simulink library "speedgoatlib_fpga_analog_io"  (R2024b)
settings: Solver=VariableStepAuto  StartTime=0.0  StopTime=10.0  RelTol=1e-3
undefined symbols (not defined in the file): IO336, sg_fpga_callBackInit_m_a1, sg_fpga_io324_analog_input_m, sg_fpga_io324_analog_output_m, sg_fpga_io324_analog_setup_m, sg_fpga_io325_analog_input_m, sg_fpga_io325_analog_output_m, sg_fpga_io325_analog_setup_m, sg_fpga_io334_analog_input_m, sg_fpga_io334_analog_output_m, sg_fpga_io334_analog_setup_m, sg_fpga_io336_analog_input_m, sg_fpga_io336_analog_output_m, sg_fpga_io336_analog_setup_m, sg_fpga_io337_analog_input_m, sg_fpga_io337_analog_output_m, sg_fpga_io337_analog_setup_m, sg_fpga_io3xx_120_analog_input_m, sg_fpga_io3xx_120_analog_output_m, sg_fpga_io3xx_120_analog_setup_m
(part 4 of 4)

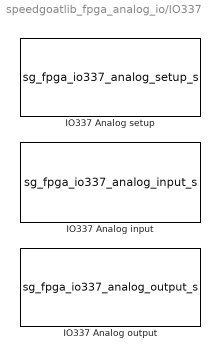
== system speedgoatlib_fpga_analog_io/IO337 ==
  IO337 Analog input : S-Function  InitFcn=sg_fpga_io337_analog_input_m.runInitFcn();  FunctionName=sg_fpga_io337_analog_input_s  Parameters=id, parSampleTime, parAiChannels, parAiChannelsStreamed, parAiReadPrevValue, parAiEnableFrame, parAiFrameSize  SFunctionDeploymentMode=off  EnableBusSupport=off  mask(ad_fpga_IO337){id=1, parSampleTime=-1, pciSlot=[-1,-1], parAiChannels=[1 2], parAiChannelsStreamed=[1 2], parAiTriggerMode=[2 2], parAiReadPrevValue=0, parAiEnableFrame=0, parAdcCoupling=[1 1 1 1], parAdcContSampling=0, parAdcDmaEnable=0, parAdcActiveDmaDevices=[1 1 1 1], parAiFrameSize=100}
      mask prompts: id "Configurable I/O Module ID"; parSampleTime "Sample Time [s]"
      mask help: Speedgoat Driver Block<br>IO337-650k - IO337 Analog Input<br><br>&copy; 2007 - 2026, Speedgoat GmbH, <a href="matlab: web('www.speedgoat.com','-browser');">www.speedgoat.com</a>
      mask init:
      | sg_fpga_io337_analog_input_m.runMaskInit();
      mask Help: eval('sg.utils.help.show(''io_main/refentry_io337_analog_input_v1'');')
      mask TypeOptions id: 1 | 2 | 3 | 4 | 5 | 6 | 7 | 8 | 9 | 10
      mask Display: disp('Speedgoat\nIO337-650k\n Analog input v1\nModule ID: 1');port_label('output',1,'1');port_label('output',2,'2');
  IO337 Analog output : S-Function  InitFcn=sg_fpga_io337_analog_output_m.runInitFcn();  FunctionName=sg_fpga_io337_analog_output_s  Parameters=id, parSampleTime, parAoChannels, parAoVoltageRange, parAoInitValues, parAoReset, parAoEnableFrame, parAoFrameSize  SFunctionDeploymentMode=off  EnableBusSupport=off  mask(da_fpga_IO337){id=1, parSampleTime=-1, pciSlot=[-1,-1], board=IO336-325k, parAoChannels=[1 2], parAoVoltageRange=[1 1], parDacOverRange=[0 0 0 0 0 0 0 0], parAoInitValues=[0 0], parAoReset=[1 1], parDacSyncOut=1, parAoEnableFrame=0, parDacActiveDmaDevices=[1 1 1 1], parDacDmaLatency=2, parAoFrameSize=1000}
      mask prompts: id "Configurable I/O Module ID"; parSampleTime "Sample Time [s]"
      mask help: Speedgoat Driver Block<br>IO337-650k - IO337 Analog output<br><br>&copy; 2007 - 2026, Speedgoat GmbH, <a href="matlab: web('www.speedgoat.com','-browser');">www.speedgoat.com</a>
      mask init:
      | sg_fpga_io337_analog_output_m.runMaskInit();
      mask Help: eval('sg.utils.help.show(''io_main/refentry_io337_analog_output_v1'');')
      mask TypeOptions id: 1 | 2 | 3 | 4 | 5 | 6 | 7 | 8 | 9 | 10
      mask Display: disp('Speedgoat\nIO337-650k\n Analog output v1\nModule ID: 1');port_label('input',1,'1');port_label('input',2,'2');
  IO337 Analog setup : S-Function  InitFcn=sg_fpga_io337_analog_setup_m.runInitFcn();  FunctionName=sg_fpga_io337_analog_setup_s  Parameters=id, p.AdcActiveChannels, p.AdcFilterWidthPow2, p.AdcOversamplRate, p.AdcDisableSampleRead, parAdcAutoCorrection, p.AdcTriggerMode, p.AdcClockDivider, p.AdcInternalTrigger, p.AdcExternalTrigger, p.AdcEnableFrame, p.AdcFrameSize, p.DacChannels, p.DacVoltageRange, p.DacInitValues, p.DacReset, parDacAutoCorrection, p.DacTriggerMode, p.DacClockDivider, p.DacInternalTrigger, p.DacExternalTrigger, p.DacEnableFrame, p.DacFifoThreshold, p.DacSourceSelection, p.EnableTriggerForCm, p.DacUsesTimer  SFunctionModules=sg_fpga_analog_dma sg_AnalogInputCm_IO334 sg_AnalogOutputCm_IO334  SFunctionDeploymentMode=off  EnableBusSupport=off  mask(analog_setup_fpga_IO337){id=1, siteIdx=1, parEnableCodeModule1=off, parEnableCodeModule2=off, parEnableCodeModule3=off, parEnableCodeModule4=off, parEnableCodeModule5=off, parEnableCodeModule6=off, parEnableCodeModule7=off, parEnableCodeModule8=off, parAdcEnableIndividualTrigger=off, parAdcDisableSampleRead=on, parAdcTriggerMode1=Model Step, parAdcSampleRate1=1e5, parAdcDioTriggerChannel1=1, parAdcInternalTrigger1=<empty>, parAdcOversampling1=None, parAdcTriggerMode2=Model Step, parAdcSampleRate2=1e5, parAdcDioTriggerChannel2=1, parAdcInternalTrigger2=<empty>, parAdcOversampling2=None, parAdcTriggerMode3=Model Step, parAdcSampleRate3=1e5, parAdcDioTriggerChannel3=1, parAdcInternalTrigger3=<empty>, parAdcOversampling3=None, parAdcTriggerMode4=Model Step, parAdcSampleRate4=1e5, parAdcDioTriggerChannel4=1, parAdcInternalTrigger4=<empty>, parAdcOversampling4=None, parAdcReadPrevValueIndividualTrigger=off, parAdcEnableFrame=off, parAdcTriggerMode=I/O Module Clock, parAdcReadPrevValue=on, parAdcSampleRate=100e3, parAdcDioTriggerChannel=1, parAdcInternalTrigger=<empty>, parAdcOversampling=None, parAdcTriggerResolution=1e-08, parAdcSampleRateFrame=1e5, parAdcFrameSize=100, parAdcSampleTime=-1, parDacTriggerMode=Model Step, parDacInternalTrigger=<empty>, parDacDioTriggerChannel=1, parDacEnableFrame=on, dacUsesTimer=on, parDacFifoThreshold=100, parDacTriggerResolution=1e-08, parDacSampleRate=1e6, parDacFrameSize=1000, parDacSampleTime=-1, parAdcChannel1=on, parAdcChannel2=on, parAdcChannel3=off, parAdcChannel4=off, parAdcChannel5=off, parAdcChannel6=off, parAdcChannel7=off, parAdcChannel8=off, parAdcAutoCorrection=on, parDacChannel1=on, parDacChannel2=on, parDacChannel3=off, parDacChannel4=off, parDacChannel5=off, parDacChannel6=off, parDacChannel7=off, parDacChannel8=off, parDacChannel9=off, parDacChannel10=off, parDacChannel11=off, parDacChannel12=off, parDacChannel13=off, parDacChannel14=off, parDacChannel15=off, parDacChannel16=off, parDacChannel17=off, parDacChannel18=off, parDacChannel19=off, parDacChannel20=off, parDacChannel21=off, parDacChannel22=off, parDacChannel23=off, parDacChannel24=off, parDacChannel25=off, parDacChannel26=off, parDacChannel27=off, parDacChannel28=off, parDacChannel29=off, parDacChannel30=off, parDacChannel31=off, parDacChannel32=off, parDacEnbIndividualSettings=on, parDacRangeCommon=+-10 V, parDacInitValueCommon=0, parDacResetCommon=on, parDacRange1=+-10 V, parDacInitValue1=0, parDacReset1=on, parDacRange2=+-10 V, parDacInitValue2=0, parDacReset2=on, parDacRange3=+-10 V, parDacInitValue3=0, parDacReset3=on, parDacRange4=+-10 V, parDacInitValue4=0, parDacReset4=on, parDacRange5=+-10 V, parDacInitValue5=0, parDacReset5=on, parDacRange6=+-10 V, parDacInitValue6=0, parDacReset6=on, parDacRange7=+-10 V, parDacInitValue7=0, parDacReset7=on, parDacRange8=+-10 V, parDacInitValue8=0, parDacReset8=on, parDacRange9=+-10 V, parDacInitValue9=0, parDacReset9=on, parDacRange10=+-10 V, parDacInitValue10=0, parDacReset10=on, parDacRange11=+-10 V, parDacInitValue11=0, parDacReset11=on, parDacRange12=+-10 V, parDacInitValue12=0, parDacReset12=on, parDacRange13=+-10 V, parDacInitValue13=0, parDacReset13=on, parDacRange14=+-10 V, parDacInitValue14=0, parDacReset14=on, parDacRange15=+-10 V, parDacInitValue15=0, parDacReset15=on, parDacRange16=+-10 V, parDacInitValue16=0, parDacReset16=on, parDacRange17=+-10 V, parDacInitValue17=0, parDacReset17=on, parDacRange18=+-10 V, parDacInitValue18=0, parDacReset18=on, parDacRange19=+-10 V, parDacInitValue19=0, parDacReset19=on, parDacRange20=+-10 V, parDacInitValue20=0, parDacReset20=on, parDacRange21=+-10 V, parDacInitValue21=0, parDacReset21=on, parDacRange22=+-10 V, parDacInitValue22=0, parDacReset22=on, parDacRange23=+-10 V, parDacInitValue23=0, parDacReset23=on, parDacRange24=+-10 V, parDacInitValue24=0, parDacReset24=on, parDacRange25=+-10 V, parDacInitValue25=0, parDacReset25=on, parDacRange26=+-10 V, parDacInitValue26=0, parDacReset26=on, parDacRange27=+-10 V, parDacInitValue27=0, parDacReset27=on, parDacRange28=+-10 V, parDacInitValue28=0, parDacReset28=on, parDacRange29=+-10 V, parDacInitValue29=0, parDacReset29=on, parDacRange30=+-10 V, parDacInitValue30=0, parDacReset30=on, parDacRange31=+-10 V, parDacInitValue31=0, parDacReset31=on, parDacRange32=+-10 V, parDacInitValue32=0, parDacReset32=on, parDacAutoCorrection=on}
      mask prompts: id "Configurable I/O Module ID"; siteIdx "Site Idx"; parAdcEnableIndividualTrigger "Enable Individual Trigger Settings"; parAdcDisableSampleRead "Disable Sample and Read"; parAdcTriggerMode1 "ADC Sample Trigger"; parAdcSampleRate1 "ADC Sample Rate [Hz]"; parAdcDioTriggerChannel1 "Digital I/O Channel"; parAdcInternalTrigger1 "Internal Signal"; parAdcOversampling1 "Oversampling Factor"; parAdcTriggerMode2 "ADC Sample Trigger"; parAdcSampleRate2 "ADC Sample Rate [Hz]"; parAdcDioTriggerChannel2 "Digital I/O Channel"; parAdcInternalTrigger2 "Internal Signal"; parAdcOversampling2 "Oversampling Factor"; parAdcTriggerMode3 "ADC Sample Trigger"; parAdcSampleRate3 "ADC Sample Rate [Hz]"; parAdcDioTriggerChannel3 "Digital I/O Channel"; parAdcInternalTrigger3 "Internal Signal"; parAdcOversampling3 "Oversampling Factor"; parAdcTriggerMode4 "ADC Sample Trigger"; parAdcSampleRate4 "ADC Sample Rate [Hz]"; parAdcDioTriggerChannel4 "Digital I/O Channel"; parAdcInternalTrigger4 "Internal Signal"; parAdcOversampling4 "Oversampling Factor"; parAdcReadPrevValueIndividualTrigger "Read Value From Previous Model Step"; parAdcEnableFrame "Enable DMA Interrupt"; parAdcTriggerMode "ADC Sample Trigger"; parAdcReadPrevValue "Read Value From Previous Model Step"; parAdcSampleRate "ADC Sample Rate [Hz]"; parAdcDioTriggerChannel "Digital I/O Channel"; parAdcInternalTrigger "Internal Signal"; parAdcOversampling "Oversampling Factor"; parAdcTriggerResolution "Trigger Resolution [s]"; parAdcSampleRateFrame "ADC Sample Rate [Hz]"; parAdcFrameSize "Frame Size (samples/channel)"; parAdcSampleTime "Input Block Sample Time [s]"; parDacTriggerMode "DAC Sample Trigger"; parDacInternalTrigger "Internal Signal"; parDacDioTriggerChannel "Digital I/O Channel"; parDacEnableFrame "Enable DMA Interrupt"; dacUsesTimer "Set Sampling Frequency"; parDacFifoThreshold "FIFO Threshold (samples/channel)"; parDacTriggerResolution "Trigger Resolution [s]"; parDacSampleRate "DAC Sample Rate [Hz]"; parDacFrameSize "Frame Size (samples/channel)"; parDacSampleTime "Output Block Sample Time [s]"; parAdcChannel1 "Ch 01"; parAdcChannel2 "Ch 02"; parAdcChannel3 "Ch 03"; parAdcChannel4 "Ch 04"; parAdcChannel5 "Ch 05"; parAdcChannel6 "Ch 06"; parAdcChannel7 "Ch 07"; parAdcChannel8 "Ch 08"; parAdcAutoCorrection "Automatic Data Correction (for Debugging)"; parDacChannel1 "Ch 1"; parDacChannel2 "Ch 2"; parDacChannel3 "Ch 3"; parDacChannel4 "Ch 4"; parDacChannel5 "Ch 5"; parDacChannel6 "Ch 6"; parDacChannel7 "Ch 7"; parDacChannel8 "Ch 8"; parDacChannel9 "Ch 9"; parDacChannel10 "Ch 10"; parDacChannel11 "Ch 11"; parDacChannel12 "Ch 12"; parDacChannel13 "Ch 13"; parDacChannel14 "Ch 14"; parDacChannel15 "Ch 15"; parDacChannel16 "Ch 16"; parDacChannel17 "Ch 17"; parDacChannel18 "Ch 18"; parDacChannel19 "Ch 19"; parDacChannel20 "Ch 20"; parDacChannel21 "Ch 21"; parDacChannel22 "Ch 22"; parDacChannel23 "Ch 23"; parDacChannel24 "Ch 24"; parDacChannel25 "Ch 25"; parDacChannel26 "Ch 26"; parDacChannel27 "Ch 27"; parDacChannel28 "Ch 28"; parDacChannel29 "Ch 29"; parDacChannel30 "Ch 30"; parDacChannel31 "Ch 31"; parDacChannel32 "Ch 32"; parDacEnbIndividualSettings "Enable individual channel settings"; parDacRangeCommon "Output Range"; parDacInitValueCommon "Initial Value [V]"; parDacResetCommon "Reset to Initial Value"; parDacRange1 "Output Range"; parDacInitValue1 "Initial Value [V]"; parDacReset1 "Reset to Initial Value"; parDacRange2 "Output Range"; parDacInitValue2 "Initial Value [V]"; parDacReset2 "Reset to Initial Value"; parDacRange3 "Output Range"; parDacInitValue3 "Initial Value [V]"; parDacReset3 "Reset to Initial Value"; parDacRange4 "Output Range"; parDacInitValue4 "Initial Value [V]"; parDacReset4 "Reset to Initial Value"; parDacRange5 "Output Range"; parDacInitValue5 "Initial Value [V]"; parDacReset5 "Reset to Initial Value"; parDacRange6 "Output Range"; parDacInitValue6 "Initial Value [V]"; parDacReset6 "Reset to Initial Value"; parDacRange7 "Output Range"; parDacInitValue7 "Initial Value [V]"; parDacReset7 "Reset to Initial Value"; parDacRange8 "Output Range"; parDacInitValue8 "Initial Value [V]"; parDacReset8 "Reset to Initial Value"; parDacRange9 "Output Range"; parDacInitValue9 "Initial Value [V]"; parDacReset9 "Reset to Initial Value"; parDacRange10 "Output Range"; parDacInitValue10 "Initial Value [V]"; parDacReset10 "Reset to Initial Value"; parDacRange11 "Output Range"; parDacInitValue11 "Initial Value [V]"; parDacReset11 "Reset to Initial Value"; parDacRange12 "Output Range"; parDacInitValue12 "Initial Value [V]"; parDacReset12 "Reset to Initial Value"; parDacRange13 "Output Range"; parDacInitValue13 "Initial Value [V]"; parDacReset13 "Reset to Initial Value"; parDacRange14 "Output Range"; parDacInitValue14 "Initial Value [V]"; parDacReset14 "Reset to Initial Value"; parDacRange15 "Output Range"; parDacInitValue15 "Initial Value [V]"; parDacReset15 "Reset to Initial Value"; parDacRange16 "Output Range"; parDacInitValue16 "Initial Value [V]"; parDacReset16 "Reset to Initial Value"; parDacRange17 "Output Range"; parDacInitValue17 "Initial Value [V]"; parDacReset17 "Reset to Initial Value"; parDacRange18 "Output Range"; parDacInitValue18 "Initial Value [V]"; parDacReset18 "Reset to Initial Value"; parDacRange19 "Output Range"; parDacInitValue19 "Initial Value [V]"; parDacReset19 "Reset to Initial Value"; parDacRange20 "Output Range"; parDacInitValue20 "Initial Value [V]"; parDacReset20 "Reset to Initial Value"; parDacRange21 "Output Range"; parDacInitValue21 "Initial Value [V]"; parDacReset21 "Reset to Initial Value"; parDacRange22 "Output Range"; parDacInitValue22 "Initial Value [V]"; parDacReset22 "Reset to Initial Value"; parDacRange23 "Output Range"; parDacInitValue23 "Initial Value [V]"; parDacReset23 "Reset to Initial Value"; parDacRange24 "Output Range"; parDacInitValue24 "Initial Value [V]"; parDacReset24 "Reset to Initial Value"; parDacRange25 "Output Range"; parDacInitValue25 "Initial Value [V]"; parDacReset25 "Reset to Initial Value"; parDacRange26 "Output Range"; parDacInitValue26 "Initial Value [V]"; parDacReset26 "Reset to Initial Value"; parDacRange27 "Output Range"; parDacInitValue27 "Initial Value [V]"; parDacReset27 "Reset to Initial Value"; parDacRange28 "Output Range"; parDacInitValue28 "Initial Value [V]"; parDacReset28 "Reset to Initial Value"; parDacRange29 "Output Range"; parDacInitValue29 "Initial Value [V]"; parDacReset29 "Reset to Initial Value"; parDacRange30 "Output Range"; parDacInitValue30 "Initial Value [V]"; parDacReset30 "Reset to Initial Value"; parDacRange31 "Output Range"; parDacInitValue31 "Initial Value [V]"; parDacReset31 "Reset to Initial Value"; parDacRange32 "Output Range"; parDacInitValue32 "Initial Value [V]"; parDacReset32 "Reset to Initial Value"; parDacAutoCorrection "Automatic Data Correction (for Debugging)"
      mask help: Speedgoat Driver Block<br>IO337-650k - IO337 Analog setup<br><br>&copy; 2007 - 2026, Speedgoat GmbH, <a href="matlab: web('www.speedgoat.com','-browser');">www.speedgoat.com</a>
      mask init:
      | p = sg_fpga_io337_analog_setup_m.runMaskInit();
      settings: OpenFcn=sg_fpga_io3xx_120_analog_setup_m.runOpenMaskCb();
      mask Help: eval('sg.utils.help.show(''io_main/refentry_io337_analog_setup_v1'');')
      mask TypeOptions id: 1 | 2 | 3 | 4 | 5 | 6 | 7 | 8 | 9 | 10
      mask TypeOptions siteIdx: 1 | 2
      mask Callback parEnableCodeModule1: sg_fpga_io337_analog_setup_m.runEnableCmCb(1);
      mask Callback parEnableCodeModule2: sg_fpga_io337_analog_setup_m.runEnableCmCb(2);
      mask Callback parEnableCodeModule3: sg_fpga_io337_analog_setup_m.runEnableCmCb(3);
      mask Callback parEnableCodeModule4: sg_fpga_io337_analog_setup_m.runEnableCmCb(4);
      mask Callback parEnableCodeModule5: sg_fpga_io337_analog_setup_m.runEnableCmCb(5);
      mask Callback parEnableCodeModule6: sg_fpga_io337_analog_setup_m.runEnableCmCb(6);
      mask Callback parEnableCodeModule7: sg_fpga_io337_analog_setup_m.runEnableCmCb(7);
      mask Callback parEnableCodeModule8: sg_fpga_io337_analog_setup_m.runEnableCmCb(8);
      mask Callback parAdcEnableIndividualTrigger: sg_fpga_io337_analog_setup_m.runAnalogInputCb();
      mask Callback parAdcDisableSampleRead: sg_fpga_io337_analog_setup_m.runAnalogInputCb();
      mask TypeOptions parAdcTriggerMode1: Model Step | I/O Module Clock | I/O Module Internal Signal | I/O Module Digital I/O
      mask Callback parAdcTriggerMode1: sg_fpga_io337_analog_setup_m.runAdcTriggerCb('suffix', '1');
      mask TypeOptions parAdcInternalTrigger1: <empty>
      mask TypeOptions parAdcOversampling1: None | 2 | 4 | 8 | 16 | 32 | 64
      mask TypeOptions parAdcTriggerMode2: Model Step | I/O Module Clock | I/O Module Internal Signal | I/O Module Digital I/O
      mask Callback parAdcTriggerMode2: sg_fpga_io337_analog_setup_m.runAdcTriggerCb('suffix', '2');
      mask TypeOptions parAdcInternalTrigger2: <empty>
      mask TypeOptions parAdcOversampling2: None | 2 | 4 | 8 | 16 | 32 | 64
      mask TypeOptions parAdcTriggerMode3: Model Step | I/O Module Clock | I/O Module Internal Signal | I/O Module Digital I/O
      mask Callback parAdcTriggerMode3: sg_fpga_io337_analog_setup_m.runAdcTriggerCb('suffix', '3');
      mask TypeOptions parAdcInternalTrigger3: <empty>
      mask TypeOptions parAdcOversampling3: None | 2 | 4 | 8 | 16 | 32 | 64
      mask TypeOptions parAdcTriggerMode4: Model Step | I/O Module Clock | I/O Module Internal Signal | I/O Module Digital I/O
      mask Callback parAdcTriggerMode4: sg_fpga_io337_analog_setup_m.runAdcTriggerCb('suffix', '4');
      mask TypeOptions parAdcInternalTrigger4: <empty>
      mask TypeOptions parAdcOversampling4: None | 2 | 4 | 8 | 16 | 32 | 64
      mask Callback parAdcEnableFrame: sg_fpga_io337_analog_setup_m.runEnableFrameCb();
      mask TypeOptions parAdcTriggerMode: Model Step | I/O Module Clock | I/O Module Internal Signal | I/O Module Digital I/O
      mask Callback parAdcTriggerMode: sg_fpga_io337_analog_setup_m.runAdcTriggerCb();
      mask TypeOptions parAdcInternalTrigger: <empty>
      mask TypeOptions parAdcOversampling: None | 2 | 4 | 8 | 16 | 32 | 64
      mask TypeOptions parDacTriggerMode: Model Step | I/O Module Clock | I/O Module Internal Signal | I/O Module Digital I/O
      mask Callback parDacTriggerMode: sg_fpga_io337_analog_setup_m.runDacTriggerCb();
      mask TypeOptions parDacInternalTrigger: <empty>
      mask Callback parDacEnableFrame: sg_fpga_io337_analog_setup_m.runDacTriggerCb();
      mask Callback dacUsesTimer: sg_fpga_io337_analog_setup_m.runDacTriggerCb();
      mask Callback parAdcChannel1: sg_fpga_io337_analog_setup_m.runAnalogInputCb();
      mask Callback parAdcChannel2: sg_fpga_io337_analog_setup_m.runAnalogInputCb();
      mask Callback parAdcChannel3: sg_fpga_io337_analog_setup_m.runAnalogInputCb();
      mask Callback parAdcChannel4: sg_fpga_io337_analog_setup_m.runAnalogInputCb();
      mask Callback parAdcChannel5: sg_fpga_io337_analog_setup_m.runAnalogInputCb();
      mask Callback parAdcChannel6: sg_fpga_io337_analog_setup_m.runAnalogInputCb();
      mask Callback parAdcChannel7: sg_fpga_io337_analog_setup_m.runAnalogInputCb();
      mask Callback parAdcChannel8: sg_fpga_io337_analog_setup_m.runAnalogInputCb();
      mask Callback parDacChannel1: sg_fpga_io337_analog_setup_m.runAnalogOutputCb();
      mask Callback parDacChannel2: sg_fpga_io337_analog_setup_m.runAnalogOutputCb();
      mask Callback parDacChannel3: sg_fpga_io337_analog_setup_m.runAnalogOutputCb();
      mask Callback parDacChannel4: sg_fpga_io337_analog_setup_m.runAnalogOutputCb();
      mask Callback parDacChannel5: sg_fpga_io337_analog_setup_m.runAnalogOutputCb();
      mask Callback parDacChannel6: sg_fpga_io337_analog_setup_m.runAnalogOutputCb();
      mask Callback parDacChannel7: sg_fpga_io337_analog_setup_m.runAnalogOutputCb();
      mask Callback parDacChannel8: sg_fpga_io337_analog_setup_m.runAnalogOutputCb();
      mask Callback parDacChannel9: sg_fpga_io337_analog_setup_m.runAnalogOutputCb();
      mask Callback parDacChannel10: sg_fpga_io337_analog_setup_m.runAnalogOutputCb();
      mask Callback parDacChannel11: sg_fpga_io337_analog_setup_m.runAnalogOutputCb();
      mask Callback parDacChannel12: sg_fpga_io337_analog_setup_m.runAnalogOutputCb();
      mask Callback parDacChannel13: sg_fpga_io337_analog_setup_m.runAnalogOutputCb();
      mask Callback parDacChannel14: sg_fpga_io337_analog_setup_m.runAnalogOutputCb();
      mask Callback parDacChannel15: sg_fpga_io337_analog_setup_m.runAnalogOutputCb();
      mask Callback parDacChannel16: sg_fpga_io337_analog_setup_m.runAnalogOutputCb();
      mask Callback parDacChannel17: sg_fpga_io337_analog_setup_m.runAnalogOutputCb();
      mask Callback parDacChannel18: sg_fpga_io337_analog_setup_m.runAnalogOutputCb();
      mask Callback parDacChannel19: sg_fpga_io337_analog_setup_m.runAnalogOutputCb();
      mask Callback parDacChannel20: sg_fpga_io337_analog_setup_m.runAnalogOutputCb();
      mask Callback parDacChannel21: sg_fpga_io337_analog_setup_m.runAnalogOutputCb();
      mask Callback parDacChannel22: sg_fpga_io337_analog_setup_m.runAnalogOutputCb();
      mask Callback parDacChannel23: sg_fpga_io337_analog_setup_m.runAnalogOutputCb();
      mask Callback parDacChannel24: sg_fpga_io337_analog_setup_m.runAnalogOutputCb();
      mask Callback parDacChannel25: sg_fpga_io337_analog_setup_m.runAnalogOutputCb();
      mask Callback parDacChannel26: sg_fpga_io337_analog_setup_m.runAnalogOutputCb();
      mask Callback parDacChannel27: sg_fpga_io337_analog_setup_m.runAnalogOutputCb();
      mask Callback parDacChannel28: sg_fpga_io337_analog_setup_m.runAnalogOutputCb();
      mask Callback parDacChannel29: sg_fpga_io337_analog_setup_m.runAnalogOutputCb();
      mask Callback parDacChannel30: sg_fpga_io337_analog_setup_m.runAnalogOutputCb();
      mask Callback parDacChannel31: sg_fpga_io337_analog_setup_m.runAnalogOutputCb();
      mask Callback parDacChannel32: sg_fpga_io337_analog_setup_m.runAnalogOutputCb();
      mask Callback parDacEnbIndividualSettings: sg_fpga_io337_analog_setup_m.runAnalogOutputCb();
      mask TypeOptions parDacRangeCommon: +-2.5 V | +-5 V | +-10 V
      mask TypeOptions parDacRange1: +-2.5 V | +-5 V | +-10 V
      mask TypeOptions parDacRange2: +-2.5 V | +-5 V | +-10 V
      mask TypeOptions parDacRange3: +-2.5 V | +-5 V | +-10 V
      mask TypeOptions parDacRange4: +-2.5 V | +-5 V | +-10 V
      mask TypeOptions parDacRange5: +-2.5 V | +-5 V | +-10 V
      mask TypeOptions parDacRange6: +-2.5 V | +-5 V | +-10 V
      mask TypeOptions parDacRange7: +-2.5 V | +-5 V | +-10 V
      mask TypeOptions parDacRange8: +-2.5 V | +-5 V | +-10 V
      mask TypeOptions parDacRange9: +-2.5 V | +-5 V | +-10 V
      mask TypeOptions parDacRange10: +-2.5 V | +-5 V | +-10 V
      mask TypeOptions parDacRange11: +-2.5 V | +-5 V | +-10 V
      mask TypeOptions parDacRange12: +-2.5 V | +-5 V | +-10 V
      mask TypeOptions parDacRange13: +-2.5 V | +-5 V | +-10 V
      mask TypeOptions parDacRange14: +-2.5 V | +-5 V | +-10 V
      mask TypeOptions parDacRange15: +-2.5 V | +-5 V | +-10 V
      mask TypeOptions parDacRange16: +-2.5 V | +-5 V | +-10 V
      mask TypeOptions parDacRange17: +-2.5 V | +-5 V | +-10 V
      mask TypeOptions parDacRange18: +-2.5 V | +-5 V | +-10 V
      mask TypeOptions parDacRange19: +-2.5 V | +-5 V | +-10 V
      mask TypeOptions parDacRange20: +-2.5 V | +-5 V | +-10 V
      mask TypeOptions parDacRange21: +-2.5 V | +-5 V | +-10 V
      mask TypeOptions parDacRange22: +-2.5 V | +-5 V | +-10 V
      mask TypeOptions parDacRange23: +-2.5 V | +-5 V | +-10 V
      mask TypeOptions parDacRange24: +-2.5 V | +-5 V | +-10 V
      mask TypeOptions parDacRange25: +-2.5 V | +-5 V | +-10 V
      mask TypeOptions parDacRange26: +-2.5 V | +-5 V | +-10 V
      mask TypeOptions parDacRange27: +-2.5 V | +-5 V | +-10 V
      mask TypeOptions parDacRange28: +-2.5 V | +-5 V | +-10 V
      mask TypeOptions parDacRange29: +-2.5 V | +-5 V | +-10 V
      mask TypeOptions parDacRange30: +-2.5 V | +-5 V | +-10 V
      mask TypeOptions parDacRange31: +-2.5 V | +-5 V | +-10 V
      mask TypeOptions parDacRange32: +-2.5 V | +-5 V | +-10 V
      mask DialogControl tabMain Prompt: Main
      mask DialogControl boxModuleSettings Prompt: Module Settings
      mask DialogControl boxCodeModules Prompt: Code Module Functionality
      mask DialogControl boxAdcTrigger Prompt: Analog Input Settings
      mask DialogControl boxAdcIndividualTrigger Prompt: Individual Trigger Settings (Sample Based)
      mask DialogControl boxAdcTrigger1 Prompt: Channel 01-02
      mask DialogControl boxAdcTrigger2 Prompt: Channel 03-04
      mask DialogControl boxAdcTrigger3 Prompt: Channel 05-06
      mask DialogControl boxAdcTrigger4 Prompt: Channel 07-08
      mask DialogControl boxAdcCommonTrigger Prompt: Common Trigger Settings
      mask DialogControl boxAdcFrameSettings Prompt: Frame-Based Settings
      mask DialogControl parAdcTriggerResolutionInfo Prompt: placeholder
      mask DialogControl parAdcSampleRateFrameInfo Prompt:
      | => 100 kHz
      | (10 us/sample)
      mask DialogControl parAdcFrameSizeInfo Prompt: => 100
      mask DialogControl parAdcSampleTimeInfo Prompt: => 1 ms
      mask DialogControl boxDacTrigger Prompt: Analog Output Trigger
      mask DialogControl boxDacFrameSettings Prompt: Frame-Based Settings
      mask DialogControl parDacFifoThresholdInfo Prompt: placeholder
      mask DialogControl parDacTriggerResolutionInfo Prompt: placeholder
      mask DialogControl parDacSampleRateInfo Prompt:
      | => 1 MHz
      | (1 us/sample)
      mask DialogControl parDacFrameSizeInfo Prompt: => 1000
      mask DialogControl parDacSampleTimeInfo Prompt: => 1 ms
      mask DialogControl tabAdc Prompt: Analog Inputs
      mask DialogControl boxAdc1 Prompt: Channel 01-08
      mask DialogControl tabDac Prompt: Analog Outputs
      mask DialogControl boxAoChannels Prompt: Available Channels
      mask DialogControl boxDacSetting Prompt: Channel Settings
      mask DialogControl boxDacCommon Prompt: Common
      mask DialogControl boxDacChannel1 Prompt: Channel 1
      mask DialogControl boxDacChannel2 Prompt: Channel 2
      mask DialogControl boxDacChannel3 Prompt: Channel 3
      mask DialogControl boxDacChannel4 Prompt: Channel 4
      mask DialogControl boxDacChannel5 Prompt: Channel 5
      mask DialogControl boxDacChannel6 Prompt: Channel 6
      mask DialogControl boxDacChannel7 Prompt: Channel 7
      mask DialogControl boxDacChannel8 Prompt: Channel 8
      mask DialogControl boxDacChannel9 Prompt: Channel 9
      mask DialogControl boxDacChannel10 Prompt: Channel 10
      mask DialogControl boxDacChannel11 Prompt: Channel 11
      mask DialogControl boxDacChannel12 Prompt: Channel 12
      mask DialogControl boxDacChannel13 Prompt: Channel 13
      mask DialogControl boxDacChannel14 Prompt: Channel 14
      mask DialogControl boxDacChannel15 Prompt: Channel 15
      mask DialogControl boxDacChannel16 Prompt: Channel 16
      mask DialogControl boxDacChannel17 Prompt: Channel 17
      mask DialogControl boxDacChannel18 Prompt: Channel 18
      mask DialogControl boxDacChannel19 Prompt: Channel 19
      mask DialogControl boxDacChannel20 Prompt: Channel 20
      mask DialogControl boxDacChannel21 Prompt: Channel 21
      mask DialogControl boxDacChannel22 Prompt: Channel 22
      mask DialogControl boxDacChannel23 Prompt: Channel 23
      mask DialogControl boxDacChannel24 Prompt: Channel 24
      mask DialogControl boxDacChannel25 Prompt: Channel 25
      mask DialogControl boxDacChannel26 Prompt: Channel 26
      mask DialogControl boxDacChannel27 Prompt: Channel 27
      mask DialogControl boxDacChannel28 Prompt: Channel 28
      mask DialogControl boxDacChannel29 Prompt: Channel 29
      mask DialogControl boxDacChannel30 Prompt: Channel 30
      mask DialogControl boxDacChannel31 Prompt: Channel 31
      mask DialogControl boxDacChannel32 Prompt: Channel 32
      mask Display: disp('Speedgoat\nIO337-650k\nAnalog setup v1\nModule ID: 1');

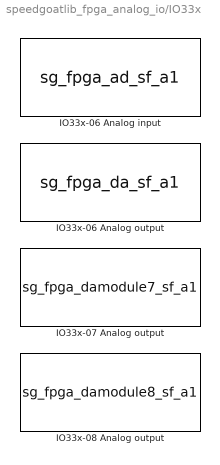
== system speedgoatlib_fpga_analog_io/IO33x ==
  IO33x-06 Analog input : S-Function  InitFcn=sg_fpga_callBackInit_m_a1;  FunctionName=sg_fpga_ad_sf_a1  Parameters="chan, trigger, range, ts,  id"  SFunctionDeploymentMode=off  EnableBusSupport=off  mask(ad_fpga_a1){id=1, chan=[1,2], range=+-10 V, trigger=Initiator, ts=0.001}
      mask prompts: id "Configurable I/O Module ID"; chan "Channel vector:"; range "Analog input range:"; trigger "Inter-module synchronization:"; ts "Sample time:"
      mask help: Speedgoat Driver Block<br>IO33x - Analog IO33x-06 Input<br><br>&copy; 2007 - 2026, Speedgoat GmbH, <a href="matlab: web('www.speedgoat.com','-browser');">www.speedgoat.com</a>
      mask init:
      | sg_fpga_ad_m_a1(id);
      mask Help: eval('sg.utils.help.show(''io_main/refentry_analog_io33x_06_input_v1'');')
      mask TypeOptions id: 1 | 2 | 3 | 4 | 5 | 6 | 7 | 8 | 9 | 10
      mask TypeOptions range: +-10 V | +-5 V | +-2.5 V | +-1.25 V
      mask TypeOptions trigger: Initiator | Target
      mask Display: disp('Speedgoat\nIO33x\nA/D read v1\nModule ID: 1');port_label('output', 1, '1');port_label('output', 2, '2');
  IO33x-06 Analog output : S-Function  InitFcn=sg_fpga_callBackInit_m_a1;  FunctionName=sg_fpga_da_sf_a1  Parameters=id, chan, trigger, initVal, resetVal, ts  SFunctionDeploymentMode=off  EnableBusSupport=off  mask(da_fpga_a1){id=1, chan=[1,2], trigger=Initiator, initVal=0, resetVal=0, ts=0.001}
      mask prompts: id "Configurable I/O Module ID"; chan "Channel vector:"; trigger "Inter-module synchronization:"; initVal "Initial Values"; resetVal "Reset to Initial Values on model stop"; ts "Sample time:"
      mask help: Speedgoat Driver Block<br>IO33x - Analog IO33x-06 Output<br><br>&copy; 2007 - 2026, Speedgoat GmbH, <a href="matlab: web('www.speedgoat.com','-browser');">www.speedgoat.com</a>
      mask init:
      | [initVal, resetVal] = sg_fpga_da_m_a1(id);
      mask Help: eval('sg.utils.help.show(''io_main/refentry_analog_io33x_06_output_v1'');')
      mask TypeOptions id: 1 | 2 | 3 | 4 | 5 | 6 | 7 | 8 | 9 | 10
      mask TypeOptions trigger: Initiator | Target
      mask Display: disp('Speedgoat\nIO33x\nD/A write v1\nModule ID: 1');port_label('input', 1, '1');port_label('input', 2, '2');
  IO33x-07 Analog output : S-Function  InitFcn=sg_fpga_callBackInit_m_a1;  FunctionName=sg_fpga_damodule7_sf_a1  Parameters="boardType, id, chan, updateMode, spiChannel, selectWord, span, initVal, resetVal,  ts, pciSlot"  SFunctionDeploymentMode=off  EnableBusSupport=off  mask(damodule7_fpga){id=1, chan=[1,2], updateMode=[0], spiChannel=[1], selectWord=[1], span=Bipolar -10V to 10V, initVal=0, resetVal=0, ts=0.001, pciSlot=-1, board=Please select...}
      mask prompts: id "Configurable I/O Module ID"; chan "Channel vector:"; updateMode "Update mode vector (0: PCI, 1: SPI):"; spiChannel "SPI channel (1-16):"; selectWord "Position in the SPI frame (1-16):"; initVal "Initial Values"; resetVal "Reset to Initial Values on model stop"; ts "Sample time:"; pciSlot "PCI slot (-1: autosearch):"
      mask help: Speedgoat Driver Block<br>IO33x - Analog IO33x-07 Output<br><br>&copy; 2007 - 2025, Speedgoat GmbH, <a href="matlab: web('www.speedgoat.com','-browser');">www.speedgoat.com</a>
      mask init:
      | [boardType, updateMode, spiChannel, selectWord, initVal, resetVal, ts] = sg_fpga_damodule7_m_a1(id, updateMode, spiChannel, selectWord, span, initVal, resetVal, ts);
      mask Help: eval('sg.utils.help.show(''io_main/refentry_analog_io33x_07_output_v1'');')
      mask TypeOptions id: 1 | 2 | 3 | 4 | 5 | 6 | 7 | 8 | 9 | 10
      mask TypeOptions span: Unipolar 0V to 5V | Unipolar 0V to 10V | Bipolar-5V to 5V | Bipolar -10V to 10V | Bipolar -2.5V to 2.5V | Bipolar -2.5V to 7.5V
      mask Display: disp('Speedgoat\nIO33x\nD/A write v1\nModule ID: 1');port_label('input', 1, '1');port_label('input', 2, '2');
  IO33x-08 Analog output : S-Function  InitFcn=sg_fpga_callBackInit_m_a1;  FunctionName=sg_fpga_damodule8_sf_a1  Parameters=boardType, id, chan, updateMode, spiChannel, selectWord, initVal, resetVal, ts, pciSlot  SFunctionDeploymentMode=off  EnableBusSupport=off  mask(damodule8_fpga){id=1, chan=[1,2], updateMode=[0], spiChannel=[1], selectWord=[1], initVal=0, resetVal=1, ts=0.001, pciSlot=-1, board=Please select...}
      mask prompts: id "Configurable I/O Module ID"; chan "Channel vector:"; updateMode "Update mode vector (0: PCI, 1: SPI):"; spiChannel "SPI channel (1-8):"; selectWord "Position in the SPI frame (1-8):"; initVal "Initial Values"; resetVal "Reset to Initial Values on model stop"; ts "Sample time:"; pciSlot "PCI slot (-1: autosearch):"
      mask help: Speedgoat Driver Block<br>IO33x - Analog IO33x-08 Output<br><br>&copy; 2007 - 2025, Speedgoat GmbH, <a href="matlab: web('www.speedgoat.com','-browser');">www.speedgoat.com</a>
      mask init:
      | [boardType, updateMode, spiChannel, selectWord, initVal, resetVal, ts] = sg_fpga_damodule8_m_a1(id, updateMode, spiChannel, selectWord, initVal, resetVal, ts);
      mask Help: eval('sg.utils.help.show(''io_main/refentry_analog_io33x_08_output_v1'');')
      mask TypeOptions id: 1 | 2 | 3 | 4 | 5 | 6 | 7 | 8 | 9 | 10
      mask Callback updateMode: sg_fpga_damodule8_m_a1_display
      mask Display: disp('Speedgoat\nIO33x\nD/A write v1\nModule ID: 1');port_label('input', 1, '1');port_label('input', 2, '2');

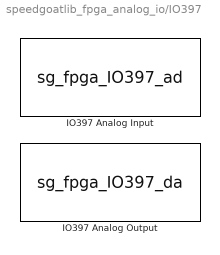
== system speedgoatlib_fpga_analog_io/IO397 ==
  IO397 Analog Input : S-Function  InitFcn=sg_fpga_callBackInit_m_a1;  FunctionName=sg_fpga_IO397_ad  Parameters=id, chan, trigger, range, ts, p.AiTriggerMode, p.AiClockDivider, parAiInternalSignal, parAiDioTriggerChannel  SFunctionDeploymentMode=off  EnableBusSupport=off  mask(ad_IO397){openMaskCallback=0, id=1, chan=[1,2], range=+5.12 V, parAiTriggerMode=I/O Module Clock, parAiInternalSignal=None, parAiDioTriggerChannel=1, parAiSampleRate=0, trigger=Initiator, ts=0.001}
      mask prompts: id "Configurable I/O Module ID"; chan "Channel vector:"; range "Analog input range:"; parAiTriggerMode "ADC Sample Trigger"; parAiInternalSignal "Internal Signal"; parAiDioTriggerChannel "Digital I/O Channel"; parAiSampleRate "ADC Sample Rate [Hz]"; trigger "Inter-module synchronization:"; ts "Sample time:"
      mask help: Speedgoat Driver Block<br>IO397-50k - Analog IO397 Input<br><br>&copy; 2007 - 2026, Speedgoat GmbH, <a href="matlab: web('www.speedgoat.com','-browser');">www.speedgoat.com</a>
      mask init:
      | p = sg_fpga_ad_io397.runMaskInit(id);
      mask Help: eval('sg.utils.help.show(''io_main/refentry_analog_io397_input_v1'');')
      mask Callback openMaskCallback: sg_fpga_ad_io397.runOpenMaskCb();
      mask TypeOptions id: 1 | 2 | 3 | 4 | 5 | 6 | 7 | 8 | 9 | 10
      mask TypeOptions range: +5.12 V | +-5 V | +-5.12 V | +10 V | +10.24 V | +-10 V | +-10.24 V
      mask TypeOptions parAiTriggerMode: Model Step | I/O Module Clock | I/O Module Internal Signal | I/O Module Digital I/O
      mask Callback parAiTriggerMode: sg_fpga_ad_io397.parTriggerMode_callback();
      mask TypeOptions parAiInternalSignal: None
      mask TypeOptions trigger: Initiator | Target
      mask DialogControl boxAnalogInputTrigger Prompt: Analog Input Trigger
      mask Display: disp('Speedgoat\nIO397-50k\nA/D read v1\nModule ID: 1');port_label('output', 1, '1');port_label('output', 2, '2');
  IO397 Analog Output : S-Function  InitFcn=sg_fpga_callBackInit_m_a1;  FunctionName=sg_fpga_IO397_da  Parameters=id, chan, initVal, resetVal, ts, span  SFunctionDeploymentMode=off  EnableBusSupport=off  mask(da_IO397){id=1, chan=[1,2], initVal=0, resetVal=0, ts=0.001, span=+-10 V}
      mask prompts: id "Configurable I/O Module ID"; chan "Channel vector:"; initVal "Initial Values"; resetVal "Reset to Initial Values on model stop"; ts "Sample time:"; span "Analog Output Range"
      mask help: Speedgoat Driver Block<br>IO397-50k - Analog IO397 Output<br><br>&copy; 2007 - 2026, Speedgoat GmbH, <a href="matlab: web('www.speedgoat.com','-browser');">www.speedgoat.com</a>
      mask init:
      | [initVal, resetVal] = sg_fpga_da_m_IO397(id);
      mask Help: eval('sg.utils.help.show(''io_main/refentry_analog_io397_output_v1'');')
      mask TypeOptions id: 1 | 2 | 3 | 4 | 5 | 6 | 7 | 8 | 9 | 10
      mask TypeOptions span: +-10 V | +-5 V | +5 V | +10 V | +10.8 V | +-10.8 V
      mask Display: disp('Speedgoat\nIO397-50k\nD/A write v1\nModule ID: 1');port_label('input', 1, '1');port_label('input', 2, '2');
